simulink model "LED"  (R2018a)
settings: Solver=FixedStepDiscrete  StartTime=0.0  StopTime=10.0  FixedStep=1/10000  RelTol=1e-3
libraries: GPIO_Lib x5, STM32_Config_Lib x1
settings Model: Creator=zqx  LastModifiedBy=zqx
settings DataIOCC: SaveFormat=Array
settings OptimizationCC: DefaultParameterBehavior=Inlined  UseDivisionForNetSlopeComputation=on  UseFloatMulNetSlope=on  InlineInvariantSignals=on  PassReuseOutputArgsAs=Individual arguments  ZeroExternalMemoryAtStartup=off  ZeroInternalMemoryAtStartup=off  NoFixptDivByZeroProtection=on  EfficientFloat2IntCast=on  LifeSpan=1  OptimizeBlockOrder=speed  DifferentSizesBufferReuse=on
settings DebuggingCC: ParameterTunabilityLossMsg=error
settings HardwareCC: ProdBitPerPointer=32  ProdBitPerSizeT=32  ProdBitPerPtrDiffT=32  ProdLargestAtomicInteger=Integer  ProdWordSize=32  ProdHWDeviceType=STMicroelectronics->STM32 32-bit Cortex-M
settings SFSimCC: MATLABDynamicMemAlloc=off
settings RTWCC: SystemTargetFile=stm32.tlc  TemplateMakefile=stm32.tmf  Description=stm32 (Embedded Target)  GenerateReport=on  IncludeHyperlinkInReport=on  LaunchReport=on  GenerateTraceInfo=on  GenerateTraceReport=on  GenerateTraceReportSl=on  GenerateTraceReportSf=on  GenerateTraceReportEml=on  GenerateWebview=on  GenerateCodeMetricsReport=on
settings CodeAppCC: ForceParamTrailComments=on  IgnoreCustomStorageClasses=off  MaxIdLength=64  OperatorAnnotations=on  SimulinkDataObjDesc=on  SFDataObjDesc=on  CustomSymbolStrGlobalVar=rt$N$M  CustomSymbolStrType=$N$M  CustomSymbolStrFcn=$N$M$F  CustomSymbolStrMacro=$N$M  InsertBlockDesc=on  ReqsInCode=on
settings STFCustomTargetCC: TargetLangStandard=C99 (ISO)  CodeReplacementLibrary=ARM CMSIS SIN COS  MultiwordLength=256  ParMdlRefBuildCompliant=on  IncludeMdlTerminateFcn=off  CombineOutputUpdateFcns=on  CombineSignalStateStructs=on  ERTCustomFileBanners=on  SupportAbsoluteTime=off  SupportNonFinite=off  SupportComplex=off  SupportContinuousTime=off  RemoveResetFunc=on  MATLABClassNameForMDSCustomization=Simulink.SoftwareTarget.ERTCustomization  GRTInterface=off  SystemTargetFile=stm32.tlc
settings ERTTargetCC: TargetLangStandard=C99 (ISO)  CodeReplacementLibrary=ARM CMSIS SIN COS  CompOptLevelCompliant=off  ConcurrentExecutionCompliant=off  IncludeMdlTerminateFcn=off  CombineSignalStateStructs=on  SupportAbsoluteTime=off  SupportNonFinite=off  SupportComplex=off  SupportNonInlinedSFcns=on  ModelStepFunctionPrototypeControlCompliant=off  CPPClassGenCompliant=off  UseToolchainInfoCompliant=off  ExtModeStaticAllocSize=256  ExtModeMexArgs=0,1,115200,10  InlinedParameterPlacement=NonHierarchical  ERTSrcFileBannerTemplate=sourceFileTemplate.cgt  ERTHdrFileBannerTemplate=sourceFileTemplate.cgt  ERTDataSrcFileTemplate=sourceFileTemplate.cgt  ERTDataHdrFileTemplate=sourceFileTemplate.cgt  ERTCustomFileTemplate=customRoutineProcess.tlc  ERTFilePackagingFormat=CompactWithDataFile

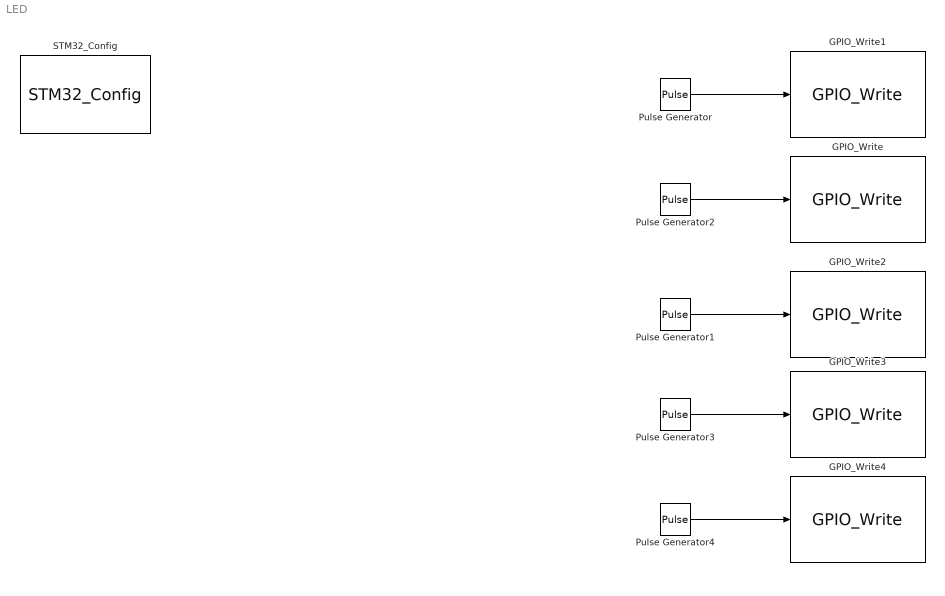
== system LED ==
  GPIO_Write : GPIO_Lib/GPIO_Write  Port_name=GPIOA  Pin0=off  Toggle_Pin0=off  Pin1=off  Toggle_Pin1=off  Pin2=off  Toggle_Pin2=off  Pin3=off  Toggle_Pin3=off  Pin4=off  Toggle_Pin4=off  Pin5=off  Toggle_Pin5=off  Pin6=off  Toggle_Pin6=off  Pin7=off  Toggle_Pin7=off  Pin8=off  Toggle_Pin8=off  Pin9=on  Toggle_Pin9=off  Pin10=off  Toggle_Pin10=off  Pin11=off  Toggle_Pin11=off  Pin12=off  Toggle_Pin12=off  Pin13=off  Toggle_Pin13=off  Pin14=off  Toggle_Pin14=off  Pin15=off  Toggle_Pin15=off  PinList="GPIOA8   9  10  11  12"
      settings: SourceProductName=Target Support Package - STM32 Adapter
  GPIO_Write1 : GPIO_Lib/GPIO_Write  Port_name=GPIOA  Pin0=off  Toggle_Pin0=off  Pin1=off  Toggle_Pin1=off  Pin2=off  Toggle_Pin2=off  Pin3=off  Toggle_Pin3=off  Pin4=off  Toggle_Pin4=off  Pin5=off  Toggle_Pin5=off  Pin6=off  Toggle_Pin6=off  Pin7=off  Toggle_Pin7=off  Pin8=on  Toggle_Pin8=off  Pin9=off  Toggle_Pin9=off  Pin10=off  Toggle_Pin10=off  Pin11=off  Toggle_Pin11=off  Pin12=off  Toggle_Pin12=off  Pin13=off  Toggle_Pin13=off  Pin14=off  Toggle_Pin14=off  Pin15=off  Toggle_Pin15=off  PinList="GPIOA8   9  10  11  12"
      settings: SourceProductName=Target Support Package - STM32 Adapter
  GPIO_Write2 : GPIO_Lib/GPIO_Write  Port_name=GPIOA  Pin0=off  Toggle_Pin0=off  Pin1=off  Toggle_Pin1=off  Pin2=off  Toggle_Pin2=off  Pin3=off  Toggle_Pin3=off  Pin4=off  Toggle_Pin4=off  Pin5=off  Toggle_Pin5=off  Pin6=off  Toggle_Pin6=off  Pin7=off  Toggle_Pin7=off  Pin8=off  Toggle_Pin8=off  Pin9=off  Toggle_Pin9=off  Pin10=on  Toggle_Pin10=off  Pin11=off  Toggle_Pin11=off  Pin12=off  Toggle_Pin12=off  Pin13=off  Toggle_Pin13=off  Pin14=off  Toggle_Pin14=off  Pin15=off  Toggle_Pin15=off  PinList="GPIOA8   9  10  11  12"
      settings: SourceProductName=Target Support Package - STM32 Adapter
  GPIO_Write3 : GPIO_Lib/GPIO_Write  Port_name=GPIOA  Pin0=off  Toggle_Pin0=off  Pin1=off  Toggle_Pin1=off  Pin2=off  Toggle_Pin2=off  Pin3=off  Toggle_Pin3=off  Pin4=off  Toggle_Pin4=off  Pin5=off  Toggle_Pin5=off  Pin6=off  Toggle_Pin6=off  Pin7=off  Toggle_Pin7=off  Pin8=off  Toggle_Pin8=off  Pin9=off  Toggle_Pin9=off  Pin10=off  Toggle_Pin10=off  Pin11=on  Toggle_Pin11=off  Pin12=off  Toggle_Pin12=off  Pin13=off  Toggle_Pin13=off  Pin14=off  Toggle_Pin14=off  Pin15=off  Toggle_Pin15=off  PinList="GPIOA8   9  10  11  12"
      settings: SourceProductName=Target Support Package - STM32 Adapter
  GPIO_Write4 : GPIO_Lib/GPIO_Write  Port_name=GPIOA  Pin0=off  Toggle_Pin0=off  Pin1=off  Toggle_Pin1=off  Pin2=off  Toggle_Pin2=off  Pin3=off  Toggle_Pin3=off  Pin4=off  Toggle_Pin4=off  Pin5=off  Toggle_Pin5=off  Pin6=off  Toggle_Pin6=off  Pin7=off  Toggle_Pin7=off  Pin8=off  Toggle_Pin8=off  Pin9=off  Toggle_Pin9=off  Pin10=off  Toggle_Pin10=off  Pin11=off  Toggle_Pin11=off  Pin12=on  Toggle_Pin12=off  Pin13=off  Toggle_Pin13=off  Pin14=off  Toggle_Pin14=off  Pin15=off  Toggle_Pin15=off  PinList="GPIOA8   9  10  11  12"
      settings: SourceProductName=Target Support Package - STM32 Adapter
  Pulse Generator{,2..4} (4 alike) : DiscretePulseGenerator  PulseType=Time based  Period=0.25  PulseWidth=50
  Pulse Generator1 : DiscretePulseGenerator  PulseType=Time based  Period=1/4  PulseWidth=50
  STM32_Config : STM32_Config_Lib/STM32_Config  Priority=0  Project_Path=C:\Users\zqx\Desktop\MATLAB_STM32\  Config_File=MATLAB_STM32.ioc  MCU_Name=STM32F103C8Tx
      settings: SourceProductName=Target Support Package - STM32 Adapter
  wires:
  Pulse Generator/1 -> GPIO_Write1/1
  Pulse Generator1/1 -> GPIO_Write2/1
  Pulse Generator2/1 -> GPIO_Write/1
  Pulse Generator3/1 -> GPIO_Write3/1
  Pulse Generator4/1 -> GPIO_Write4/1
